simulink model "mppt_invert"  (R2016a)
settings: Solver=VariableStepAuto  StartTime=0.0  StopTime=10.0  RelTol=1e-3
values from neighbouring files (symbols this model uses):
  phase = angle(Xk)    [dft2.m]
undefined symbols (not defined in the file or in its folder): Cfmax, Lf, RLf, Tss
libraries: powerlib x10, powerlib_meascontrol x3, simulink x1, re_lib x1
settings Model: Creator=Emdadul Haq  LastModifiedBy=Emdadul Haq

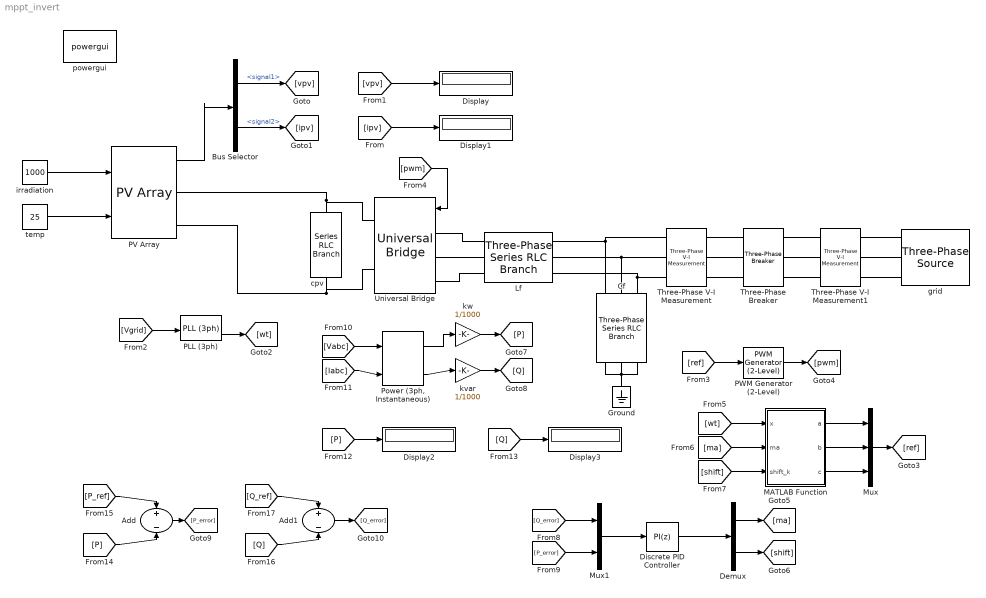
== system mppt_invert ==
  Add : Sum  Inputs=+-
  Add1 : Sum  Inputs=+-
  Bus Selector : BusSelector  OutputSignals=signal1,signal2
  Cf : powerlib/Elements/Three-Phase Series RLC Branch  LConnTagsString=A|B|C  RConnTagsString=A|B|C  BranchType=RC  Resistance=1e-6  Inductance=Lf  Capacitance=Cfmax  Measurements=None
  Demux : Demux  Outputs=2
  Discrete PID Controller : simulink/Continuous/PID Controller  Controller=PI  TimeDomain=Discrete-time  SampleTime=Tss*100  IntegratorMethod=Forward Euler  FilterMethod=Forward Euler  Form=Parallel  UseFilter=on  ControllerParametersSource=internal  P=.01  I=1  D=0  N=100  InitialConditionSource=internal  InitialConditionForIntegrator=0  InitialConditionForFilter=0  ExternalReset=none  LimitOutput=on  UpperSaturationLimit=1.1  LowerSaturationLimit=-1.1  LinearizeAsGain=off  AntiWindupMode=none  Kb=1  TrackingMode=off  Kt=1  PParamMin=[]  PParamMax=[]  IParamMin=[]  IParamMax=[]  DParamMin=[]  DParamMax=[]  NParamMin=[]  NParamMax=[]  KbParamMin=[]  KbParamMax=[]  KtParamMin=[]  KtParamMax=[]  POutMin=[]  POutMax=[]  IOutMin=[]  IOutMax=[]  DOutMin=[]  DOutMax=[]  NOutMin=[]  NOutMax=[]  KbOutMin=[]  KbOutMax=[]  KtOutMin=[]  KtOutMax=[]  IntegratorOutMin=[]  IntegratorOutMax=[]  FilterOutMin=[]  FilterOutMax=[]  SumOutMin=[]  SumOutMax=[]  SumI1OutMin=[]  SumI1OutMax=[]  SumI2OutMin=[]  SumI2OutMax=[]  SumI3OutMin=[]  SumI3OutMax=[]  SumDOutMin=[]  SumDOutMax=[]  SaturationOutMin=[]  SaturationOutMax=[]  IntegratorContinuousStateAttributes=''  IntegratorStateMustResolveToSignalObject=off  IntegratorRTWStateStorageClass=Auto  FilterContinuousStateAttributes=''  FilterStateMustResolveToSignalObject=off  FilterRTWStateStorageClass=Auto  DifferentiatorICPrevScaledInput=0  DifferentiatorOutMin=[]  DifferentiatorOutMax=[]
  Display{,1..3} (4 alike) : Display
  Ground : powerlib/Elements/Ground  LConnTagsString=a
  Lf : powerlib/Elements/Three-Phase Series RLC Branch  LConnTagsString=A|B|C  RConnTagsString=A|B|C  BranchType=RL  Resistance=RLf  Inductance=Lf  Capacitance=Lf  Measurements=None
  MATLAB Function : MATLAB Function  TreatAsAtomicUnit=on
  Mux : Mux  Inputs=3
  Mux1 : Mux  Inputs=2
  PLL (3ph) : powerlib_meascontrol/PLL/PLL (3ph)  Fmin=45  Par_Init=[0, 50]  ParK=[180, 3200, 1]  TcD=1e-4  MaxRateChangeFreq=12  FilterCutOffFreq=25  Ts=Tss  AGC=on
  PV Array : re_lib/Solar/PV Array  Npar=4  Nser=27  PlotType=array @ 25 deg.C & specified irradiances  S_vec="[ 1000  500  250 ]"  Temp_C_vec="[ 45 25  ]"  ModuleName=1Soltech 1STH-215-P  PlotWhenSelected=off  Pm=213.15  Ncell=60  Voc=36.3  Isc=7.84  Vm=29  Im=7.35  beta_Voc_pc=-0.36099  alpha_Isc_pc=0.102  beta_Voc=-0.13104  alpha_Isc=0.007997  IL=7.8649  I0=2.9259e-10  nI=0.98117  Rsh=313.3991  Rs=0.39383  BAL=on  Tc=1e-6  Tfilter=5e-5
  PWM Generator (2-Level) : powerlib_meascontrol/Pulse & Signal Generators/PWM Generator (2-Level)  ModulatorType=Three-phase bridge (6 pulses)  ModulatorMode=Unsynchronized  Fc=fsw  Pc=90  nF=27  MinMax="[ -1  1 ]"  SamplingTechnique=Natural  ModulatingSignals=off  m=0.8  Freq=60  Phase=0  Ts=Tss  ShowCarrierOutport=off
  "Power (3ph, Instantaneous)" : powerlib_meascontrol/Measurements/Power (3ph, Instantaneous)
  Three-Phase V-I Measurement : powerlib/Measurements/Three-Phase V-I Measurement  VoltageMeasurement=phase-to-ground  SetLabelV=on  LabelV=Vabc  Vpu=off  VpuLL=off  CurrentMeasurement=yes  SetLabelI=on  LabelI=Iabc  Ipu=off  Pbase=100e6  Vbase=500e3  OutputType=Complex  PhasorSimulation=off  PSBequivalent=0
  Three-Phase V-I Measurement1 : powerlib/Measurements/Three-Phase V-I Measurement  VoltageMeasurement=phase-to-ground  SetLabelV=on  LabelV=Vgrid  Vpu=off  VpuLL=off  CurrentMeasurement=yes  SetLabelI=on  LabelI=Igrid  Ipu=off  Pbase=100e6  Vbase=500e3  OutputType=Complex  PhasorSimulation=off  PSBequivalent=0
  Three-Phase Breaker : powerlib/Elements/Three-Phase Breaker  InitialState=open  SwitchA=on  SwitchB=on  SwitchC=on  SwitchTimes="[1/50  10]"  External=off  BreakerResistance=0.01  SnubberResistance=1e6  SnubberCapacitance=inf  Measurements=None
  Universal Bridge : powerlib/Power Electronics/Universal Bridge  Arms=3  SnubberResistance=1e5  SnubberCapacitance=inf  Device=IGBT / Diodes  Ron=1e-3  Lon=0  ForwardVoltages="[  0  0  ]"  ForwardVoltage=0  GTOparameters=[ 10e-6 , 20e-6 ]  IGBTparameters=[ 1e-6 , 2e-6 ]  Measurements=None  Measurements_2=None  converterType=Rectifier
  cpv : powerlib/Elements/Series RLC Branch  LConnTagsString=__new0  RConnTagsString=__new0  BranchType=RC  Resistance=1e-3  Inductance=1e-6  SetiL0=off  InitialCurrent=0  Capacitance=1000e-6  Setx0=off  InitialVoltage=0  Measurements=None
  grid : powerlib/Electrical Sources/Three-Phase Source  InternalConnection=Yg  VoltagePhases=off  Voltage=25e3  PhaseAngle=0  Voltage_phases=[25e3 25e3 25e3]/sqrt(3)  PhaseAngles_phases=[0 -120 +120]  Frequency=60  NonIdealSource=on  SpecifyImpedance=off  Resistance=0.8929  Inductance=16.58e-3  ShortCircuitLevel=100e6  BaseVoltage=25e3  XRratio=7  BusType=swing  Pref=10e3  Qref=0  Prefabc=[10e3, 10e3, 10e3]  Qrefabc=[0, 0, 0]  Qmin=-inf  Qmax=inf
  irradiation : Constant  Value=1000
  kvar : Gain  Gain=1/1000
  kw : Gain  Gain=1/1000
  powergui : powerlib/powergui  Priority=1  SimulationMode=Discrete  SolverType=Tustin/Backward Euler (TBE)  SampleTime=5e-6  frequency=60  SPID=off  DisableSnubberDevices=off  DisableRonSwitches=off  DisableVfSwitches=off  SwTol=0  DisplayEquations=off  Interpol=off  ExternalGateDelay=off  methode=off  Ts=10  FunctionMessages=off  echomessages=off  HookPort=off  EnableUseOfTLC=off  x0status=blocks  frequencyindice=0  Pbase=100e6  ErrMax=1e-4  Iterations=50  UnitsV=kV  UnitsW=MW  buscounter=0  RestoreLinks=warning  ResistiveCurrentMeasurement=off  Frange=[0:2:500]  Ylog=off  Xlog=on  ShowGrid=off  save=off  variable=ZData  structure=0  ZoomFFT=off  StartTime=0.0  cycles=1  DisplayStyle=1  fundamental=60  FreqAxis=off  MaxFrequency=1000  frequencyindicesteady=1  RmsSteady=1  display=off
  "temp " : Constant  Value=25
  wires:
  irradiation/1 -> PV Array/1
  "temp "/1 -> PV Array/2
  PV Array/1 -> Bus Selector/1
  Bus Selector/1 -> [vpv]  "<signal1>"
  Bus Selector/2 -> [ipv]  "<signal2>"
  [ipv] -> Display1/1
  [vpv] -> Display/1
  [Vgrid] -> PLL (3ph)/1
  PLL (3ph)/2 -> [wt]
  MATLAB Function/2(b) -> Mux/2
  MATLAB Function/1(a) -> Mux/1
  MATLAB Function/3(c) -> Mux/3
  Mux/1 -> [ref]
  [ref] -> PWM Generator (2-Level)/1
  PWM Generator (2-Level)/1 -> [pwm]
  [pwm] -> Universal Bridge/1
  [wt] -> MATLAB Function/1(x)
  [ma] -> MATLAB Function/2(ma)
  [shift] -> MATLAB Function/3(shift_k)
  Mux1/1 -> Discrete PID Controller/1
  Discrete PID Controller/1 -> Demux/1
  Demux/1 -> [ma]
  Demux/2 -> [shift]
  [Q_error] -> Mux1/1
  [P_error] -> Mux1/2
  [Vabc] -> "Power (3ph, Instantaneous)"/1
  [Iabc] -> "Power (3ph, Instantaneous)"/2
  "Power (3ph, Instantaneous)"/1 -> kw/1
  "Power (3ph, Instantaneous)"/2 -> kvar/1
  kw/1 -> [P]
  kvar/1 -> [Q]
  [P] -> Display2/1
  [Q] -> Display3/1
  Add/1 -> [P_error]
  [P] -> Add/2
  [P_ref] -> Add/1
  [Q] -> Add1/2
  [Q_ref] -> Add1/1
  Add1/1 -> [Q_error]
  connections:
  PV Array/RConn1 -- Universal Bridge/RConn1 -- cpv/LConn1
  PV Array/RConn2 -- Universal Bridge/RConn2 -- cpv/RConn1
  Lf/LConn1 -- Universal Bridge/LConn1
  Lf/LConn2 -- Universal Bridge/LConn2
  Universal Bridge/LConn3 -- Lf/LConn3
  Lf/RConn1 -- Cf/LConn1 -- Three-Phase V-I Measurement/LConn1
  Lf/RConn2 -- Three-Phase V-I Measurement/LConn2 -- Cf/LConn2
  Lf/RConn3 -- Three-Phase V-I Measurement/LConn3 -- Cf/LConn3
  Cf/RConn1 -- Ground/LConn1 -- Cf/RConn2 -- Cf/RConn3
  Three-Phase Breaker/LConn1 -- Three-Phase V-I Measurement/RConn1
  Three-Phase V-I Measurement/RConn2 -- Three-Phase Breaker/LConn2
  Three-Phase V-I Measurement/RConn3 -- Three-Phase Breaker/LConn3
  Three-Phase V-I Measurement1/RConn1 -- Three-Phase Breaker/RConn1
  Three-Phase V-I Measurement1/RConn2 -- Three-Phase Breaker/RConn2
  Three-Phase V-I Measurement1/RConn3 -- Three-Phase Breaker/RConn3
  grid/RConn1 -- Three-Phase V-I Measurement1/LConn1
  Three-Phase V-I Measurement1/LConn2 -- grid/RConn2
  Three-Phase V-I Measurement1/LConn3 -- grid/RConn3

== matlab function mppt_invert/MATLAB Function ==
  data: x input; a output; ma input; shift_k input; b output; c output
function [a,b,c] =ref_generation(x,ma,shift_k)
a=(ma*(sin((x)+shift_k)));
b=(ma*(sin((x)+shift_k-(2*pi/3))));
c=(ma*(sin((x)+shift_k+(2*pi/3))));
